simulink model "Missile_Guidance"  (R2025b)
settings: Solver=VariableStepAuto  StartTime=0.0  StopTime=10.0  RelTol=1e-3
libraries: simulink x1
settings Model: Creator=ahmed  LastModifiedBy=ahmed

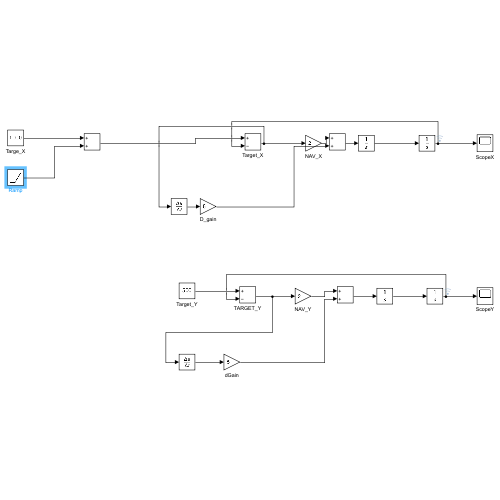
[thumbnail: Simulink's stored preview of the top-level diagram]
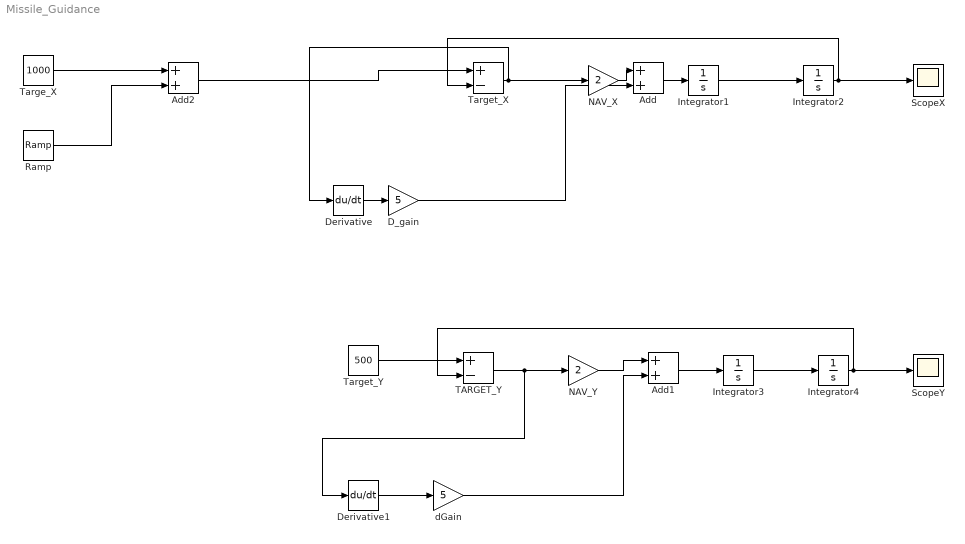
== system Missile_Guidance ==
  Add : Sum
  Add1 : Sum
  Add2 : Sum
  D_gain : Gain  Gain=5
  Derivative : Derivative
  Derivative1 : Derivative
  Integrator{1..4} (4 alike) : Integrator
  NAV_X : Gain  Gain=2
  NAV_Y : Gain  Gain=2
  Ramp : simulink/Sources/Ramp  slope=20  start=0  InitialOutput=0
  ScopeX : Scope
      settings: ActiveDisplayYMinimum=-1  ActiveDisplayYMaximum=1
  ScopeY : Scope
      settings: ActiveDisplayYMinimum=-61.542223727734566  ActiveDisplayYMaximum=553.88001354961125
  TARGET_Y : Sum  Inputs=+-
  Targe_X : Constant  Value=1000
  Target_X : Sum  Inputs=+-
  Target_Y : Constant  Value=500
  dGain : Gain  Gain=5
  wires:
  Target_X/1 -> Derivative/1, NAV_X/1
  NAV_X/1 -> Add/1
  Integrator1/1 -> Integrator2/1
  Integrator2/1 -> Target_X/2, ScopeX/1
  D_gain/1 -> Add/2
  Derivative/1 -> D_gain/1
  Add/1 -> Integrator1/1
  Target_Y/1 -> TARGET_Y/1
  TARGET_Y/1 -> Derivative1/1, NAV_Y/1
  Integrator4/1 -> TARGET_Y/2, ScopeY/1
  Integrator3/1 -> Integrator4/1
  Add1/1 -> Integrator3/1
  NAV_Y/1 -> Add1/1
  Derivative1/1 -> dGain/1
  dGain/1 -> Add1/2
  Targe_X/1 -> Add2/1
  Ramp/1 -> Add2/2
  Add2/1 -> Target_X/1
